simulink model "indMotorSpeedControl"  (R2023b)
settings: Solver=VariableStepAuto  StartTime=0.0  StopTime=10.0  RelTol=1e-3
libraries: spsControlledVoltageSourceLib x3, spsAsynchronousMachineSIUnitsLib x2, spsGroundLib x2, spsThreePhaseVIMeasurementLib x2, simulink x1, spsThreePhaseProgrammableVoltageSourceLib x1, spspowerguiLib x1
settings Model: Creator=klysm  LastModifiedBy=klysm

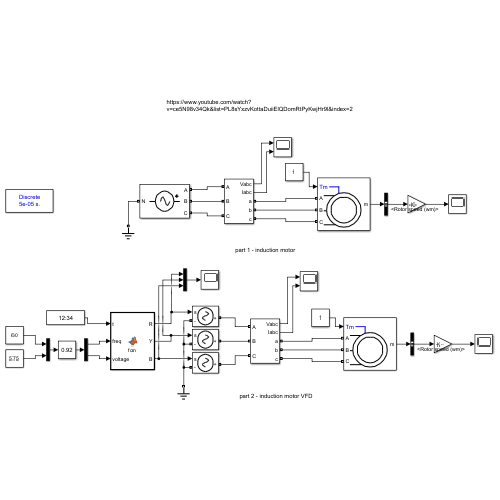
[thumbnail: Simulink's stored preview of the top-level diagram]
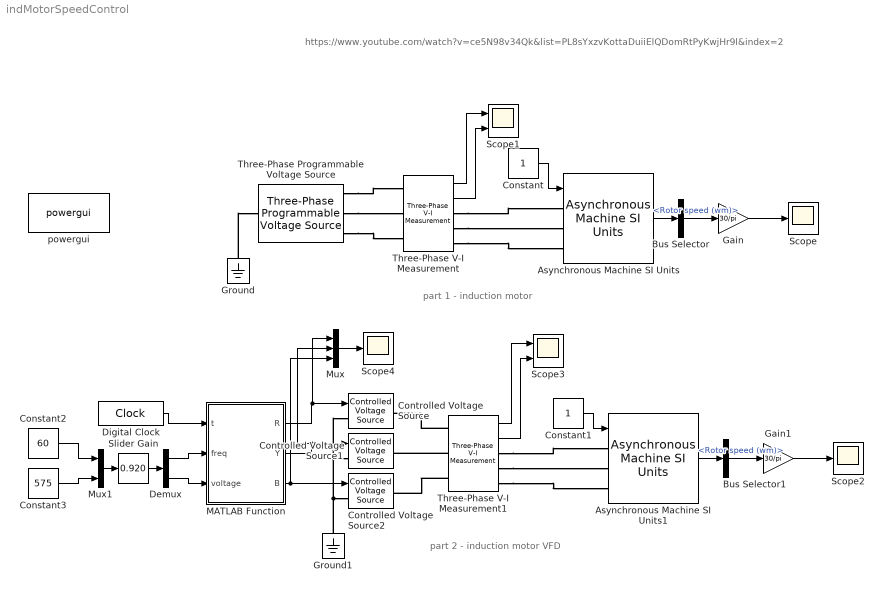
== system indMotorSpeedControl ==
  note: part 2 - induction motor VFD
  note: https://www.youtube.com/watch?v=ce5N98v34Qk&list=PL8sYxzvKottaDuiiElQDomRtPyKwjHr9l&index=2
  note: part 1 - induction motor
  Asynchronous Machine SI Units : spsAsynchronousMachineSIUnitsLib/Asynchronous Machine SI Units  RotorType=Squirrel-cage  PresetModel="14:  200 HP 575 V 60Hz 1785 RPM"  MechanicalLoad=Torque Tm  ShowDetailedParameters=on  ReferenceFrame=Rotor  Units=SI  MeasurementBus=off  NominalParameters=[1.492e+05 575 60]  VoltageRatio=1  Stator=[0.02475 0.000284]  Rotor=[0.01329 0.000284]  Cage1=[0.4155 0.002066]  Cage2=[0.4168 0.0003495]  Lm=0.01425  Mechanical=[2.6 0.06346 2]  PolePairs=2  InitialConditions=[0 0 0 0 0 0 0 0]  SimulateSaturation=off  Saturation=[14.03593122, 27.81365428, 53.79336849, 72.68890987, 97.98006896, 148.6815601, 215.7428561, 302.9841135, 428.7778367 ; 230, 322, 414, 460, 506, 552, 598, 644, 690]  LoadFlowParameters=1492000  TsPowergui=0  TsBlock=-1  IterativeModel=Trapezoidal non iterative  IterativeDiscreteModel=Trapezoidal non iterative  Pmec=1.492e+006
  Asynchronous Machine SI Units1 : spsAsynchronousMachineSIUnitsLib/Asynchronous Machine SI Units  RotorType=Squirrel-cage  PresetModel="14:  200 HP 575 V 60Hz 1785 RPM"  MechanicalLoad=Torque Tm  ShowDetailedParameters=on  ReferenceFrame=Rotor  Units=SI  MeasurementBus=off  NominalParameters=[1.492e+05 575 60]  VoltageRatio=1  Stator=[0.02475 0.000284]  Rotor=[0.01329 0.000284]  Cage1=[0.4155 0.002066]  Cage2=[0.4168 0.0003495]  Lm=0.01425  Mechanical=[2.6 0.06346 2]  PolePairs=2  InitialConditions=[0 0 0 0 0 0 0 0]  SimulateSaturation=off  Saturation=[14.03593122, 27.81365428, 53.79336849, 72.68890987, 97.98006896, 148.6815601, 215.7428561, 302.9841135, 428.7778367 ; 230, 322, 414, 460, 506, 552, 598, 644, 690]  LoadFlowParameters=1492000  TsPowergui=0  TsBlock=-1  IterativeModel=Trapezoidal non iterative  IterativeDiscreteModel=Trapezoidal non iterative  Pmec=1.492e+006
  Bus Selector : BusSelector  OutputSignals=Mechanical.Rotor speed (wm)
  Bus Selector1 : BusSelector  OutputSignals=Mechanical.Rotor speed (wm)
  Constant : Constant
  Constant1 : Constant
  Constant2 : Constant  Value=60
  Constant3 : Constant  Value=575
  Controlled Voltage Source : spsControlledVoltageSourceLib/Controlled Voltage Source  Initialize=on  Source_Type=AC  Amplitude=0  Phase=0  Frequency=0  Measurements=None
  Controlled Voltage Source1 : spsControlledVoltageSourceLib/Controlled Voltage Source  Initialize=on  Source_Type=AC  Amplitude=0  Phase=0  Frequency=0  Measurements=None
  Controlled Voltage Source2 : spsControlledVoltageSourceLib/Controlled Voltage Source  Initialize=on  Source_Type=AC  Amplitude=0  Phase=0  Frequency=0  Measurements=None
  Demux : Demux  Outputs=2
  Digital Clock : DigitalClock  SampleTime=5e-5
  Gain : Gain  Gain=30/pi
  Gain1 : Gain  Gain=30/pi
  Ground : spsGroundLib/Ground  LConnTagsString=a
  Ground1 : spsGroundLib/Ground  LConnTagsString=a
  MATLAB Function : MATLAB Function  TreatAsAtomicUnit=on
  Mux : Mux  Inputs=3
  Mux1 : Mux  Inputs=2
  Scope : Scope
  Scope1 : Scope  NumInputPorts=2
  Scope2 : Scope
  Scope3 : Scope  NumInputPorts=2
  Scope4 : Scope
  Slider Gain : simulink/Math Operations/Slider Gain  gain=0.920  low=0  high=2
  Three-Phase Programmable Voltage Source : spsThreePhaseProgrammableVoltageSourceLib/Three-Phase Programmable Voltage Source  PositiveSequence="[575  0 60]"  VariationEntity=None  VariationType=Table of time-amplitude pairs  VariationTypeAlt=Step  VariationStep=0.5  VariationRate=10  VariationMagnitude=0.3  VariationFrequency=2  VariationTiming=[1 2]  VariationPhaseA=off  Amplitudes=[1 0.8 1.2 1.0]  TimeValues=[0 0.1 0.15 0.2]  HarmonicGeneration=off  HarmonicA=[3 0.2 -25 0]  HarmonicB=[2 0.15 35 2]  Timing="[0.05  3]"  BusType=swing  Pref=0  Qref=0  Qmin=-inf  Qmax=inf
  Three-Phase V-I Measurement : spsThreePhaseVIMeasurementLib/Three-Phase V-I Measurement  VoltageMeasurement=phase-to-ground  SetLabelV=off  LabelV=Vabc  Vpu=off  VpuLL=off  CurrentMeasurement=yes  SetLabelI=off  LabelI=Iabc  Ipu=off  Pbase=100e6  Vbase=500e3  OutputType=Complex  PhasorSimulation=off  PSBequivalent=0
  Three-Phase V-I Measurement1 : spsThreePhaseVIMeasurementLib/Three-Phase V-I Measurement  VoltageMeasurement=phase-to-ground  SetLabelV=off  LabelV=Vabc  Vpu=off  VpuLL=off  CurrentMeasurement=yes  SetLabelI=off  LabelI=Iabc  Ipu=off  Pbase=100e6  Vbase=500e3  OutputType=Complex  PhasorSimulation=off  PSBequivalent=0
  powergui : spspowerguiLib/powergui  Priority=1  SimulationMode=Discrete  SampleTime=50e-6  frequency=60  Iterations=50  frequencyindice=60  Pbase=100e6  ErrMax=1e-4  UnitsV=kV  UnitsW=MW  buscounter=0  FunctionMessages=off  echomessages=off  EnableUseOfTLC=off  CurrentSourceSwitches=off  DisableSnubberDevices=off  DisableRonSwitches=off  DisableVfSwitches=off  DisplayEquations=off  AutomaticDiscreteSolvers=off  SolverType=Tustin/Backward Euler (TBE)  Interpol=off  ExternalGateDelay=off  methode=off  Ts=100  x0status=blocks  SPID=on  SwTol=0  HookPort=off  NonlinearTolerance=1e-4  nMaxIteration=100  ContinueOnMaxIteration=off  RestoreLinks=warning  ResistiveCurrentMeasurement=off  Frange=[0:2:500]  Ylog=off  Xlog=on  ShowGrid=off  save=off  variable=ZData  structure=0  ZoomFFT=off  StartTime=0.0  cycles=1  DisplayStyle=1  fundamental=60  FreqAxis=off  MaxFrequency=1000  frequencyindicesteady=1  RmsSteady=1  display=off
  wires:
  Constant/1 -> Asynchronous Machine SI Units/1
  Asynchronous Machine SI Units/1 -> Bus Selector/1
  Bus Selector/1 -> Gain/1  "<Rotor speed (wm)>"
  Gain/1 -> Scope/1
  Three-Phase V-I Measurement/1 -> Scope1/1
  Three-Phase V-I Measurement/2 -> Scope1/2
  Three-Phase V-I Measurement1/2 -> Scope3/2
  Asynchronous Machine SI Units1/1 -> Bus Selector1/1
  Gain1/1 -> Scope2/1
  Constant1/1 -> Asynchronous Machine SI Units1/1
  Bus Selector1/1 -> Gain1/1  "<Rotor speed (wm)>"
  Three-Phase V-I Measurement1/1 -> Scope3/1
  Digital Clock/1 -> MATLAB Function/1(t)
  MATLAB Function/2(Y) -> Mux/2, Controlled Voltage Source1/1
  MATLAB Function/3(B) -> Mux/3, Controlled Voltage Source2/1
  MATLAB Function/1(R) -> Mux/1, Controlled Voltage Source/1
  Mux/1 -> Scope4/1
  Mux1/1 -> Slider Gain/1
  Slider Gain/1 -> Demux/1
  Demux/1 -> MATLAB Function/2(freq)
  Demux/2 -> MATLAB Function/3(voltage)
  Constant2/1 -> Mux1/1
  Constant3/1 -> Mux1/2
  connections:
  Three-Phase Programmable Voltage Source/RConn2 -- Three-Phase V-I Measurement/LConn2
  Three-Phase Programmable Voltage Source/RConn3 -- Three-Phase V-I Measurement/LConn3
  Three-Phase Programmable Voltage Source/RConn1 -- Three-Phase V-I Measurement/LConn1
  Three-Phase V-I Measurement/RConn2 -- Asynchronous Machine SI Units/LConn2
  Three-Phase V-I Measurement/RConn1 -- Asynchronous Machine SI Units/LConn1
  Three-Phase V-I Measurement/RConn3 -- Asynchronous Machine SI Units/LConn3
  Ground/LConn1 -- Three-Phase Programmable Voltage Source/LConn1
  Three-Phase V-I Measurement1/RConn1 -- Asynchronous Machine SI Units1/LConn1
  Three-Phase V-I Measurement1/RConn3 -- Asynchronous Machine SI Units1/LConn3
  Three-Phase V-I Measurement1/LConn2 -- Controlled Voltage Source1/RConn1
  Three-Phase V-I Measurement1/LConn3 -- Controlled Voltage Source2/RConn1
  Three-Phase V-I Measurement1/LConn1 -- Controlled Voltage Source/RConn1
  Three-Phase V-I Measurement1/RConn2 -- Asynchronous Machine SI Units1/LConn2
  Ground1/LConn1 -- Controlled Voltage Source/LConn1 -- Controlled Voltage Source1/LConn1 -- Controlled Voltage Source2/LConn1

== matlab function indMotorSpeedControl/MATLAB Function ==
  data: t input; R output; freq input; voltage input; Y output; B output
function [R,Y,B] = fcn(t,freq,voltage)
omega=2*pi*freq;
R=voltage*sin(omega*t);
B=voltage*sin(omega*t+120*pi/180);
Y=voltage*sin(omega*t+240*pi/180);
